simulink model "prz_st"  (R2014b)
settings: Solver=ode45  StartTime=0.0  StopTime=Tsym  RelTol=1e-3
undefined symbols (not defined in the file): A, alfa, deltaFc, deltaFd, deltaFh, deltaTc, deltaTd, deltaTh, Fc, Fc0, Fd, Fd0, Fh, Fh0, h0, T0, tau, tauh, Tc, Tc0, Tciagly, Td, Td0, Th, Th0, Tskok
settings Model: Creator=Arek  LastModifiedBy=Arek
settings DebuggingCC: SolverPrmCheckMsg=none

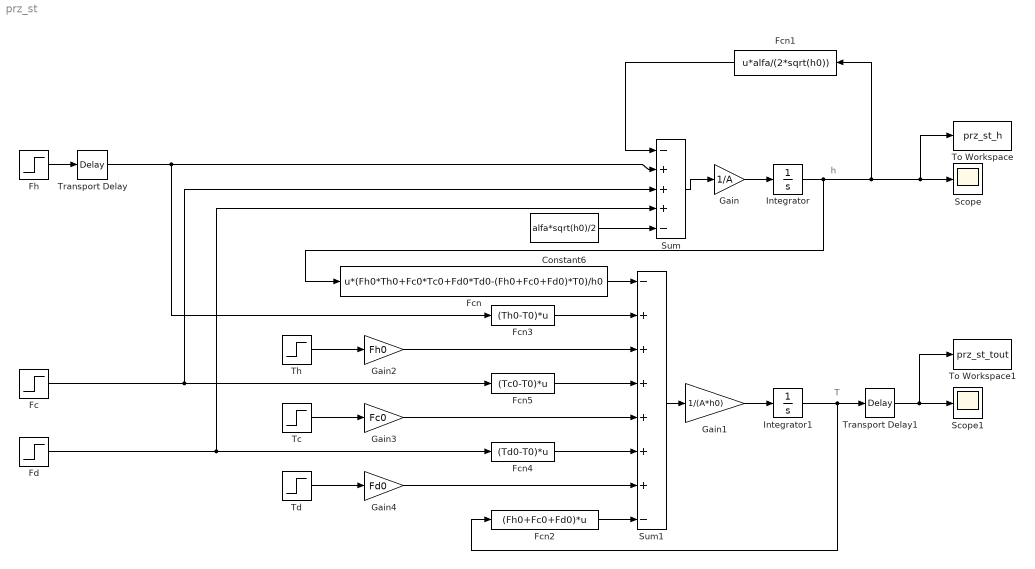
== system prz_st ==
  note: T
  note: h
  Constant6 : Constant  Value=alfa*sqrt(h0)/2
  Fc : Step  Time=Tskok  Before=Fc  After=Fc+deltaFc  SampleTime=Tciagly
  Fcn : Fcn  Expr=u*(Fh0*Th0+Fc0*Tc0+Fd0*Td0-(Fh0+Fc0+Fd0)*T0)/h0
  Fcn1 : Fcn  Expr=u*alfa/(2*sqrt(h0))
  Fcn2 : Fcn  Expr=(Fh0+Fc0+Fd0)*u
  Fcn3 : Fcn  Expr=(Th0-T0)*u
  Fcn4 : Fcn  Expr=(Td0-T0)*u
  Fcn5 : Fcn  Expr=(Tc0-T0)*u
  Fd : Step  Time=Tskok  Before=Fd  After=Fd+deltaFd  SampleTime=Tciagly
  Fh : Step  Time=Tskok  Before=Fh  After=Fh+deltaFh  SampleTime=Tciagly
  Gain : Gain  Gain=1/A
  Gain1 : Gain  Gain=1/(A*h0)
  Gain2 : Gain  Gain=Fh0
  Gain3 : Gain  Gain=Fc0
  Gain4 : Gain  Gain=Fd0
  Integrator : Integrator  InitialCondition=h0
  Integrator1 : Integrator  InitialCondition=T0
  Scope : Scope
  Scope1 : Scope
  Sum : Sum  Inputs=-+++-
  Sum1 : Sum  Inputs=-++++++-
  Tc : Step  Time=Tskok  Before=Tc  After=Tc+deltaTc  SampleTime=Tciagly
  Td : Step  Time=Tskok  Before=Td  After=Td+deltaTd  SampleTime=Tciagly
  Th : Step  Time=Tskok  Before=Th  After=Th+deltaTh  SampleTime=Tciagly
  To Workspace : ToWorkspace  VariableName=prz_st_h  SaveFormat=Timeseries  SampleTime=-1
  To Workspace1 : ToWorkspace  VariableName=prz_st_tout  SaveFormat=Timeseries  SampleTime=-1
  Transport Delay : TransportDelay  DelayTime=tauh  InitialOutput=Fh
  Transport Delay1 : TransportDelay  DelayTime=tau  InitialOutput=T0
  wires:
  Integrator1/1 -> Transport Delay1/1, Fcn2/1
  Integrator/1 -> Fcn/1, Fcn1/1, To Workspace/1, Scope/1
  Transport Delay/1 -> Sum/2, Fcn3/1
  Fc/1 -> Sum/3, Fcn5/1
  Fd/1 -> Sum/4, Fcn4/1
  Gain/1 -> Integrator/1
  Sum/1 -> Gain/1
  Fcn1/1 -> Sum/1
  Gain1/1 -> Integrator1/1
  Sum1/1 -> Gain1/1
  Fcn/1 -> Sum1/1
  Fcn2/1 -> Sum1/8
  Gain2/1 -> Sum1/3
  Th/1 -> Gain2/1
  Tc/1 -> Gain3/1
  Td/1 -> Gain4/1
  Gain4/1 -> Sum1/7
  Gain3/1 -> Sum1/5
  Fcn3/1 -> Sum1/2
  Fcn5/1 -> Sum1/4
  Fcn4/1 -> Sum1/6
  Fh/1 -> Transport Delay/1
  Transport Delay1/1 -> To Workspace1/1, Scope1/1
  Constant6/1 -> Sum/5
